simulink model "myproject_exec"  (Simulink 3.00)
libraries: execlib x7

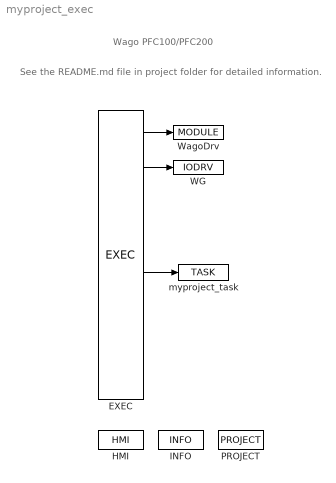
== system myproject_exec ==
  note: See the README.md file in project
      | folder for detailed information.
  note: Wago PFC100/PFC200
  EXEC : execlib/EXEC  target=Generic target device  tick=0.02  ntick0=2  ntick1=50  ntick2=100  ntick3=1200  pri0=5  pri1=9  pri2=13  pri3=18
  HMI : execlib/HMI  IncludeHMI=on  HmiDir=hmi  SourceDir=hmisrc  GenerateWebWatch=on  GenerateRexHMI=off  RedirectToHMI=off  Compression=off
  INFO : execlib/INFO  Title=Wago PFC100/PFC200 example
  PROJECT : execlib/PROJECT  SourcesOnTarget=off
  WG : execlib/IODRV  module=WagoDrv  classname=WagoDrv  factor=1  stack=10240  pri=3  timer=off
  WagoDrv : execlib/MODULE
  myproject_task : execlib/TASK  factor=1  start=0  stop=1  stack=10240  MDLOPEN=on
  wires:
  EXEC/1 -> WagoDrv/1
  EXEC/2 -> WG/1
  EXEC/5 -> myproject_task/1
